simulink model "Tire1_basic01"  (R2022a)
settings: Solver=VariableStepAuto  StartTime=0.0  StopTime=10  RelTol=1e-3
values from neighbouring files (symbols this model uses):
  Tire_MagicB = 10    [TireParam.m]
  Tire_MagicC = 1.9    [TireParam.m]
  Tire_MagicD = 0.9    [TireParam.m]
  Tire_MagicE = 0.97    [TireParam.m]
undefined symbols (not defined in the file or in its folder): sigbuilder_block
libraries: fl_lib x5, nesl_utility x4, sdl_lib x1
settings Model: Creator=amyyang  LastModifiedBy=amyyang
settings SolverCC: AlgebraicLoopSolver=TrustRegion
settings DebuggingCC: UnconnectedInputMsg=warning  UnconnectedOutputMsg=warning  UnconnectedLineMsg=warning  SFMachineParentedDataDiag=warning
settings RTWCC: DLArmComputeVersion=19.05
settings SimscapeCC: SimscapeLogType=local  SimscapeLogToSDI=on  SimscapeLogLimitData=off

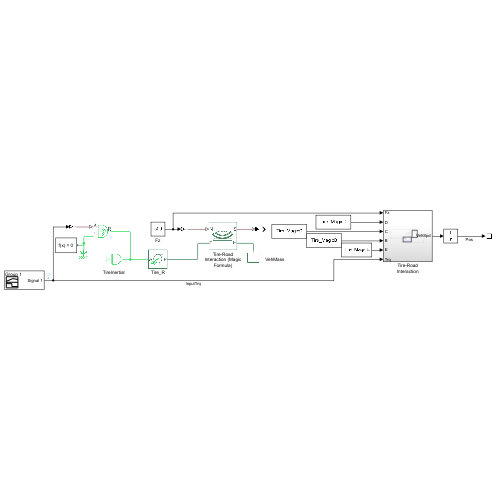
[thumbnail: Simulink's stored preview of the top-level diagram]
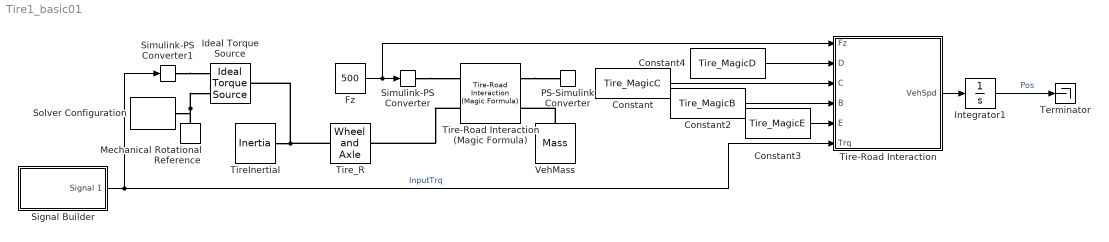
== system Tire1_basic01 ==
  Constant : Constant  Value=Tire_MagicC
  Constant2 : Constant  Value=Tire_MagicB
  Constant3 : Constant  Value=Tire_MagicE
  Constant4 : Constant  Value=Tire_MagicD
  Fz : Constant  Value=500
  Ideal Torque Source : fl_lib/Mechanical/Mechanical Sources/Ideal Torque Source
      settings: SourceProductBaseCode=PW,SS,VE
  Integrator1 : Integrator
  Mechanical Rotational Reference : fl_lib/Mechanical/Rotational Elements/Mechanical Rotational Reference
      settings: SourceProductBaseCode=PW,SS,VE
  PS-Simulink Converter : nesl_utility/PS-Simulink Converter  PhysicalDomain=network_engine_domain  SubClassName=ps_output  LeftPortType=input  RightPortType=output  PseudoPeriodic=off  Frequencies=[]  VectorFormat=1-D array  Unit=inherit  AffineConversion=off
      settings: SourceProductBaseCode=SS,PW,VE
  Signal Builder : Subsystem  Tag=STV Subsys  LoadFcn=sigbuilder_block('load');  StartFcn=sigbuilder_block('start');  StopFcn=sigbuilder_block('stop');  ClipboardFcn=sigbuilder_block('clipboard');  mask(Sigbuilder block){tuvar=[0:10]}
      mask help: Simulink:masks:SigbuilderBlock_MD
      mask init:
      | if ~strcmp(get_param(bdroot(gcbh),'SimulationStatus'),'stopped') tuvar = sigbuilder_block('maskInit'); end
      settings: CopyFcn=sigbuilder_block('copy');  DeleteFcn=sigbuilder_block('delete');  ModelCloseFcn=sigbuilder_block('modelClose');  PreSaveFcn=sigbuilder_block('preSave');  PauseFcn=sigbuilder_block('pause');  ContinueFcn=sigbuilder_block('continue');  NameChangeFcn=sigbuilder_block('namechange');  OpenFcn=sigbuilder_block('open',[437.6 199.2 550.4 400 ]);  CloseFcn=sigbuilder_block('close');
      mask Display: plot(0, 0, 100, 100,[2, 2, 32, 32, 2], [68, 8, 8, 68, 68],[32, 2], [38, 38], [32, 19, 2],[53, 60, 44], [32, 17, 17, 2],[16, 16, 31, 31]);txt = getActiveGroup(gcbh);text(2, 100, txt,'verticalAlignment', 'top');
  Simulink-PS Converter : nesl_utility/Simulink-PS Converter  PhysicalDomain=network_engine_domain  SubClassName=ps_input  LeftPortType=input  RightPortType=output  PseudoPeriodic=off  Frequencies=[]  NoiseDistribution=none  NoiseParameters=[]  Unit=1  AffineConversion=off  FilteringAndDerivatives=provide  SimscapeFilterOrder=1  InputFilterTimeConstant=0.001  UdotUserProvided=0
      settings: SourceProductBaseCode=SS,PW,VE
  Simulink-PS Converter1 : nesl_utility/Simulink-PS Converter  PhysicalDomain=network_engine_domain  SubClassName=ps_input  LeftPortType=input  RightPortType=output  PseudoPeriodic=off  Frequencies=[]  NoiseDistribution=none  NoiseParameters=[]  Unit=N*m  AffineConversion=off  FilteringAndDerivatives=provide  SimscapeFilterOrder=1  InputFilterTimeConstant=0.001  UdotUserProvided=0
      settings: SourceProductBaseCode=SS,PW,VE
  Solver Configuration : nesl_utility/Solver Configuration  PhysicalDomain=network_engine_domain  SubClassName=solver  LeftPortType=input  RightPortType=generic  Tones=[]  Harmonics=[]  SimulateNoise=off  Profile=off  UseLocalSampling=off  EnableSwitchedLinearOptims=on  FrequencyDomain=off  UseCCode=off  RelTol=0.001  AbsTol=1e-06  MinStep=1e-09  ToWorkspace=off  RevertToSquareIcSolve=off  NumHomotopyIterations=100  PhasorMode=off  PhasorModeNumHarmonics=1  IndexReductionMethod=DerivativeReplacement  DoDC=off  ResidualTolerance=1e-09  UseLocalSolver=off  LocalSolverChoice=NE_BACKWARD_EULER_ADVANCER  LocalSolverSampleTime=0.001  DoFixedCost=off  MaxNonlinIter=3  MaxModeIter=2  ComputeImpulses=off  ImpulseIterations=2  LinearAlgebra=auto  LinearAlgebraNumThread=0  EquationFormulation=NE_TIME_EF  DelaysMemoryBudget=1024  AutomaticFiltering=on  FilteringTimeConstant=0.001  PartitionStorageMethod=AS_NEEDED  PartitionMemoryBudget=1024  PartitionMethod=ROBUST
      settings: SourceProductBaseCode=SS,PW,VE
  Terminator : Terminator
  Tire-Road Interaction : Subsystem
  Tire-Road Interaction (Magic Formula) : sdl_lib/Tires & Vehicles/Tire Subcomponents/Tire-Road Interaction (Magic Formula)  parameterization=sdl.enum.magic_tire_model.constant  F_z1=3000 N  F_x1=3500 N  kappa1=10  B_m=Tire_MagicB  C_m=Tire_MagicC  D_m=Tire_MagicD  E_m=Tire_MagicE  fz0=4000 N  p_Cx=1.685  p_Dx=[1.21, -.037]  p_Ex=[.344, .095, -.02, 0]  p_Kx=[21.51, -.163, .245]  p_Hx=[-.002, .002]  p_Vx=[0, 0]  v_tr_thr=0.1 m/s
      settings: SourceProductBaseCode=LD  LogSimulationData=on  InternalSimscapePortConfiguration="{\"Bottom\":[],\"Left\":[{\"id\":\"N\",\"label\":\"N\",\"type\":\"input\"},{\"id\":\"T\",\"label\":\"T\",\"type\":\"foundation.mechanical.translational.translational\"}],\"Right\":[{\"id\":\"S\",\"label\":\"S\",\"type\":\"output\"},{\"id\":\"H\",\"label\":\"H\",\"type\":\"foundation.mechanical.translational.translational\"}],\"Top\":[]}"
  TireInertial : fl_lib/Mechanical/Rotational Elements/Inertia  inertia=1 kg*m^2  num_ports=foundation.enum.numPorts2.one  w_specify=off  w_priority=High  w=0 rad/s  w_nominal_specify=off  w_nominal_unit=rad/s  w_nominal_value=1  t_specify=off  t_priority=None  t=0 N*m  t_nominal_specify=off  t_nominal_unit=N*m  t_nominal_value=1
      settings: SourceProductBaseCode=PW,SS,VE
  Tire_R : fl_lib/Mechanical/Mechanisms/Wheel and Axle  R=0.3 m  or=1  t_specify=off  t_priority=None  t=0 N*m  t_nominal_specify=off  t_nominal_unit=N*m  t_nominal_value=1  f_specify=off  f_priority=None  f=0 N  f_nominal_specify=off  f_nominal_unit=N  f_nominal_value=1
      settings: SourceProductBaseCode=PW,SS,VE  LogSimulationData=on
  VehMass : fl_lib/Mechanical/Translational Elements/Mass  mass=50 kg  num_ports=foundation.enum.numPorts2.one  v_specify=off  v_priority=High  v=0 m/s  v_nominal_specify=off  v_nominal_unit=m/s  v_nominal_value=1  f_specify=off  f_priority=None  f=0 N  f_nominal_specify=off  f_nominal_unit=N  f_nominal_value=1
      settings: SourceProductBaseCode=PW,SS,VE  LogSimulationData=on
  wires:
  Integrator1/1 -> Terminator/1  "Pos"
  Constant4/1 -> Tire-Road Interaction/2(D)
  Constant/1 -> Tire-Road Interaction/3(C)
  Constant2/1 -> Tire-Road Interaction/4(B)
  Constant3/1 -> Tire-Road Interaction/5(E)
  Signal Builder/1(Signal 1) -> Simulink-PS Converter1/1, Tire-Road Interaction/6(Trq)  "InputTrq"
  Tire-Road Interaction/1(VehSpd) -> Integrator1/1
  Fz/1 -> Tire-Road Interaction/1(Fz), Simulink-PS Converter/1
  connections:
  Tire-Road Interaction (Magic Formula)/LConn2 -- Tire_R/RConn1
  Simulink-PS Converter/RConn1 -- Tire-Road Interaction (Magic Formula)/LConn1
  Tire-Road Interaction (Magic Formula)/RConn1 -- PS-Simulink Converter/LConn1
  VehMass/LConn1 -- Tire-Road Interaction (Magic Formula)/RConn2
  Tire_R/LConn1 -- TireInertial/LConn1 -- Ideal Torque Source/LConn1
  Simulink-PS Converter1/RConn1 -- Ideal Torque Source/RConn1
  Mechanical Rotational Reference/LConn1 -- Solver Configuration/RConn1 -- Ideal Torque Source/RConn2

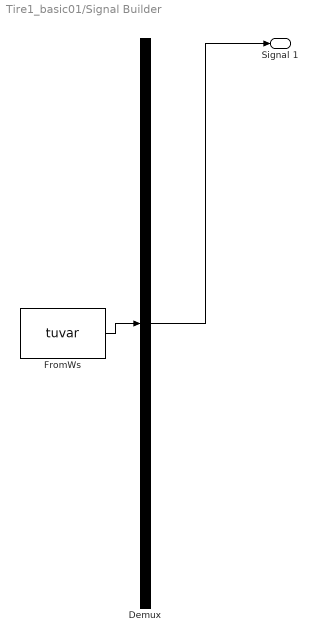
== system Tire1_basic01/Signal Builder ==
  Demux : Demux  Tag=STV Demux  Outputs=1
      settings: DisplayOption=none
  FromWs : FromWorkspace  Tag=STV FromWs  VariableName=tuvar
      SigBuilderData=|
      | common.afterFinalStr = 'Extrapolate'
      | common.sampleTime = 0
      | dataSet.timeRange = [0 10]
      | dataSet.name = 'Group 1'
      | sbobj.Groups.Name = 'Group 1'
      | sbobj.Groups.Signals.Name = 'Signal 1'
      | sbobj.Groups.Signals.XData = [0 2 4 6 8 10]
      | sbobj.Groups.Signals.YData = [0 0 150 100 0 0]
  Signal 1 : Outport  Tag=STV Outport
  wires:
  Demux/1 -> Signal 1/1
  FromWs/1 -> Demux/1

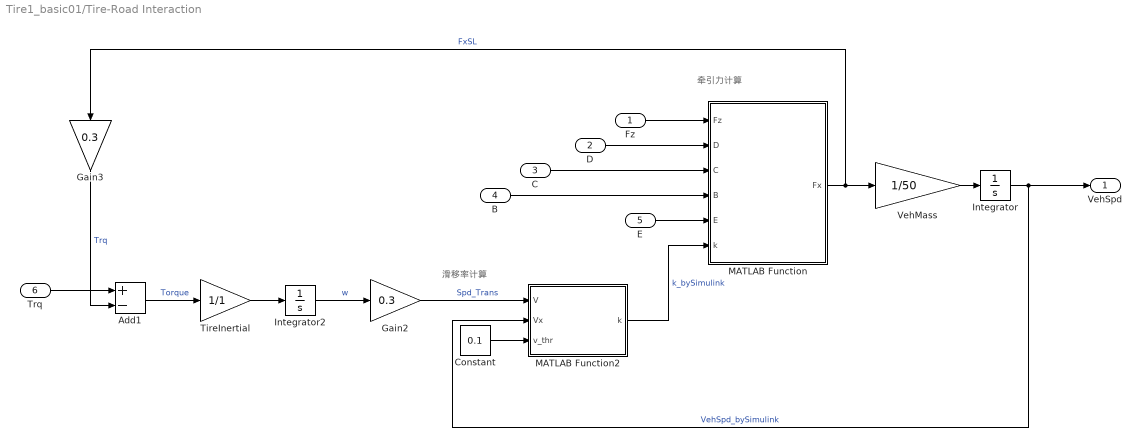
== system Tire1_basic01/Tire-Road Interaction ==
  note: 牵引力计算
  note: 滑移率计算
  Fz : Inport
  D : Inport  Port=2
  C : Inport  Port=3
  B : Inport  Port=4
  E : Inport  Port=5
  Trq : Inport  Port=6
  Add1 : Sum  Inputs=+-
  Constant : Constant  Value=0.1
  Gain2 : Gain  Gain=0.3
  Gain3 : Gain  Gain=0.3
  Integrator : Integrator
  Integrator2 : Integrator
  MATLAB Function : MATLAB Function  TreatAsAtomicUnit=on
  MATLAB Function2 : MATLAB Function  TreatAsAtomicUnit=on
  TireInertial : Gain  Gain=1/1
  VehMass : Gain  Gain=1/50
  VehSpd : Outport
  wires:
  D/1 -> MATLAB Function/2(D)
  Add1/1 -> TireInertial/1  "Torque"
  Integrator/1 -> MATLAB Function2/2(Vx), VehSpd/1  "VehSpd_bySimulink"
  MATLAB Function/1(Fx) -> Gain3/1, VehMass/1  "FxSL"
  TireInertial/1 -> Integrator2/1
  Trq/1 -> Add1/1
  VehMass/1 -> Integrator/1
  Gain2/1 -> MATLAB Function2/1(V)  "Spd_Trans"
  Fz/1 -> MATLAB Function/1(Fz)
  E/1 -> MATLAB Function/5(E)
  B/1 -> MATLAB Function/4(B)
  C/1 -> MATLAB Function/3(C)
  Integrator2/1 -> Gain2/1  "w"
  Gain3/1 -> Add1/2  "Trq"
  MATLAB Function2/1(k) -> MATLAB Function/6(k)  "k_bySimulink"
  Constant/1 -> MATLAB Function2/3(v_thr)

== matlab function Tire1_basic01/Tire-Road Interaction/MATLAB Function ==
  data: Fz input; D input; C input; B input; E input; Fx output; k input
function Fx = fcn(Fz,D,C,B,E,k)

Fx = Fz * D*sin(C*atan(B*k - E*(B*k - atan(B*k))));
end

== matlab function Tire1_basic01/Tire-Road Interaction/MATLAB Function2 ==
  data: V input; k output; Vx input; v_thr input
function k = fcn(V,Vx,v_thr)

Vsx = V - Vx; %spd slip

if abs(Vx) > abs(v_thr)
     k = Vsx/abs(Vx);
else
     k = 2*Vsx/(v_thr + Vx^2/v_thr);
     %k = 0;
end
 
 
end
